simulink model "EPLL_PFC"  (R2019b)
settings: Solver=ode45  StartTime=0.0  StopTime=1  MaxStep=1e-6  AbsTol=1e-6
values from neighbouring files (symbols this model uses):
  C = 4000e-6    (= 0.004)    [EPLL_PFC_params.m]
  E = 670    [EPLL_PFC_params.m]
  f_VT = 3700    [EPLL_PFC_params.m]
  K_vco = 1    [EPLL_PFC_params.m]
  L = (400e-6)/2    (= 0.0002)    [EPLL_PFC_params.m]
  mu_1 = 200    [EPLL_PFC_params.m]
  omega_vco_free = 50 * 2 * pi    (= 314.159265359)    [EPLL_PFC_params.m]
  R = 1.22    [EPLL_PFC_params.m]
  t_step = 1/f_VT/N1    (= 1.35135135135e-06)    [EPLL_PFC_params.m]
  tau_1 = 1/mu_2    (= 5e-05)    [EPLL_PFC_params.m]
  tau_2 = mu_3/mu_2    (= 0.02)    [EPLL_PFC_params.m]
undefined symbols (not defined in the file or in its folder): sawtooth
libraries: powerlib x15
settings Model: Creator=Vogal  LastModifiedBy=mir
settings SolverCC: AutoScaleAbsTol=off  InitialStep=1e-6
settings DataIOCC: ReturnWorkspaceOutputs=off
settings OptimizationCC: LifeSpan=inf
settings DebuggingCC: AllowSymbolicDim=off  SFExecutionAtInitializationDiag=none  ArithmeticOperatorsInVariantConditions=warning
settings HardwareCC: ProdBitPerSizeT=32  ProdBitPerPtrDiffT=32  ProdWordSize=32  ProdHWDeviceType=Specified
settings SFSimCC: SimUseLocalCustomCode=off  CustomCodeUndefinedFunction=UseInterfaceOnly
settings RTWCC: RTWUseLocalCustomCode=off
settings CodeAppCC: StateflowObjectComments=on
settings SimscapeCC: SimscapeNormalizeSystem=off

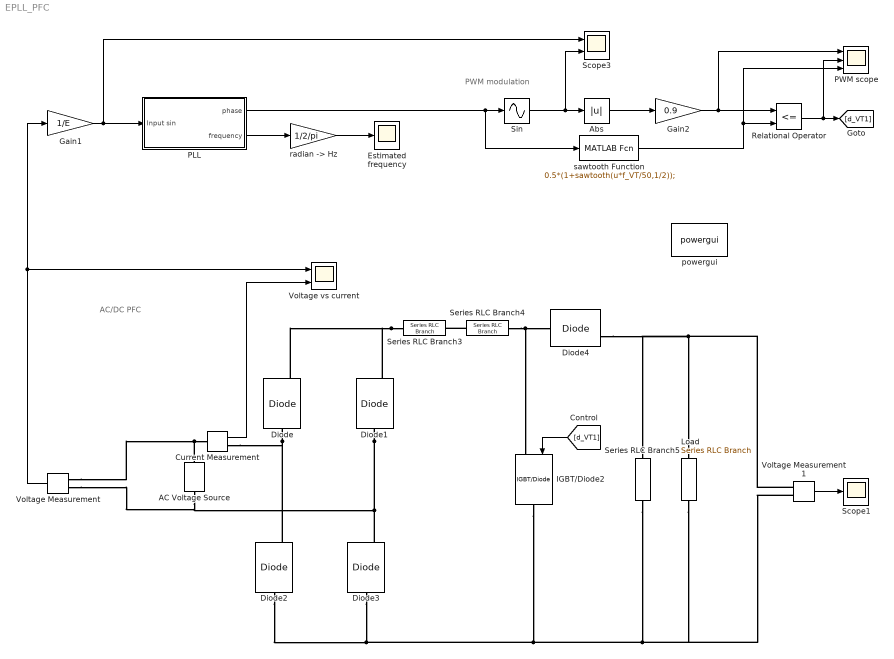
== system EPLL_PFC ==
  note: PWM modulation
  note: AC/DC PFC
  AC Voltage Source : powerlib/Electrical Sources/AC Voltage Source  Amplitude=E  Phase=0  Frequency=55  SampleTime=0  Measurements=None  BusType=swing  Pref=10e3  Qref=0  Qmin=-inf  Qmax=+inf
      settings: SourceProductName=Simscape Electrical
  Abs : Abs
  Current Measurement : powerlib/Measurements/Current Measurement  PhasorSimulation=off  OutputType=Complex  PSBequivalent=0
      settings: SourceProductName=Simscape Electrical
  Diode{,1..4} (5 alike) : powerlib/Power Electronics/Diode  Ron=0.001  Lon=0  Vf=0.8  IC=0  UseSnubber=off  Rs=500  Cs=250e-9  Measurements=on
      settings: SourceProductName=Simscape Electrical
  Estimated frequency : Scope
  Gain1 : Gain  Gain=1/E
  Gain2 : Gain  Gain=0.9
  IGBT/Diode2 : powerlib/Power Electronics/IGBT//Diode  Ron=1e-3  Rs=1e5  Cs=inf  Measurements=off
      settings: SourceProductName=Simscape Electrical
  Load : powerlib/Elements/Series RLC Branch  LConnTagsString=__new0  RConnTagsString=__new0  BranchType=R  Resistance=R  Inductance=L  SetiL0=off  InitialCurrent=0  Capacitance=C  Setx0=off  InitialVoltage=0  Measurements=None
      settings: SourceProductName=Simscape Electrical
  PLL : Subsystem
  PWM scope : Scope  NumInputPorts=3
  Relational Operator : RelationalOperator  Operator=<=  OutDataTypeStr=boolean  RndMeth=Nearest
  Scope1 : Scope
  Scope3 : Scope  NumInputPorts=2
  Series RLC Branch3 : powerlib/Elements/Series RLC Branch  LConnTagsString=__new0  RConnTagsString=__new0  BranchType=L  Resistance=R  Inductance=L  SetiL0=off  InitialCurrent=0  Capacitance=1e-6  Setx0=off  InitialVoltage=0  Measurements=None
      settings: SourceProductName=Simscape Electrical
  Series RLC Branch4 : powerlib/Elements/Series RLC Branch  LConnTagsString=__new0  RConnTagsString=__new0  BranchType=R  Resistance=1  Inductance=L  SetiL0=off  InitialCurrent=0  Capacitance=C  Setx0=off  InitialVoltage=0  Measurements=None
      settings: SourceProductName=Simscape Electrical
  Series RLC Branch5 : powerlib/Elements/Series RLC Branch  LConnTagsString=__new0  RConnTagsString=__new0  BranchType=C  Resistance=R  Inductance=L  SetiL0=off  InitialCurrent=0  Capacitance=C  Setx0=off  InitialVoltage=0  Measurements=None
      settings: SourceProductName=Simscape Electrical
  Sin : Sin  TimeSource=Use external signal  SampleTime=0
  Voltage Measurement : powerlib/Measurements/Voltage Measurement  PhasorSimulation=off  OutputType=Complex  PSBequivalent=0
      settings: SourceProductName=Simscape Electrical
  Voltage Measurement1 : powerlib/Measurements/Voltage Measurement  PhasorSimulation=off  OutputType=Complex  PSBequivalent=0
      settings: SourceProductName=Simscape Electrical
  Voltage vs current : Scope  NumInputPorts=2
  powergui : powerlib/powergui  Priority=1  SimulationMode=Discrete  SampleTime=t_step  frequency=60  Iterations=50  frequencyindice=0  Pbase=100e6  ErrMax=1e-4  UnitsV=kV  UnitsW=MW  buscounter=0  FunctionMessages=off  echomessages=off  EnableUseOfTLC=off  CurrentSourceSwitches=off  DisableSnubberDevices=off  DisableRonSwitches=off  DisableVfSwitches=off  DisplayEquations=off  AutomaticDiscreteSolvers=off  SolverType=Tustin/Backward Euler (TBE)  Interpol=off  ExternalGateDelay=off  methode=off  Ts=10  x0status=blocks  SPID=off  SwTol=0  HookPort=off  NonlinearTolerance=1e-4  nMaxIteration=100  ContinueOnMaxIteration=off  RestoreLinks=warning  ResistiveCurrentMeasurement=off  Frange=[0:2:500]  Ylog=off  Xlog=on  ShowGrid=off  save=off  variable=ZData  structure=0  ZoomFFT=off  StartTime=0.0  cycles=1  DisplayStyle=1  fundamental=60  FreqAxis=off  MaxFrequency=1000  frequencyindicesteady=1  RmsSteady=1  display=off
      settings: SourceProductName=Simscape Electrical
  "radian -> Hz" : Gain  Gain=1/2/pi
  sawtooth Function : MATLABFcn  MATLABFcn=0.5*(1+sawtooth(u*f_VT/50,1/2));
  wires:
  [d_VT1] -> IGBT/Diode2/1
  Voltage Measurement/1 -> Gain1/1, Voltage vs current/1
  Relational Operator/1 -> PWM scope/2, [d_VT1]
  Gain2/1 -> PWM scope/1, Relational Operator/1
  Current Measurement/1 -> Voltage vs current/2
  Voltage Measurement1/1 -> Scope1/1
  Abs/1 -> Gain2/1
  Gain1/1 -> Scope3/1, PLL/1("Input sin ")
  PLL/1(phase) -> sawtooth Function/1, Sin/1
  sawtooth Function/1 -> PWM scope/3, Relational Operator/2
  PLL/2(frequency) -> "radian -> Hz"/1
  "radian -> Hz"/1 -> Estimated frequency/1
  Sin/1 -> Scope3/2, Abs/1
  connections:
  Diode3/LConn1 -- Diode2/LConn1 -- Load/RConn1 -- Voltage Measurement1/LConn2 -- Series RLC Branch5/RConn1 -- IGBT/Diode2/RConn1
  Diode/LConn1 -- Diode2/RConn1 -- Current Measurement/RConn1
  Series RLC Branch5/LConn1 -- Diode4/RConn1 -- Load/LConn1 -- Voltage Measurement1/LConn1
  Series RLC Branch4/LConn1 -- IGBT/Diode2/LConn1 -- Diode4/LConn1
  Series RLC Branch3/LConn1 -- Diode/RConn1 -- Diode1/RConn1
  Diode1/LConn1 -- Voltage Measurement/LConn2 -- AC Voltage Source/LConn1 -- Diode3/RConn1
  Series RLC Branch4/RConn1 -- Series RLC Branch3/RConn1
  AC Voltage Source/RConn1 -- Voltage Measurement/LConn1 -- Current Measurement/LConn1

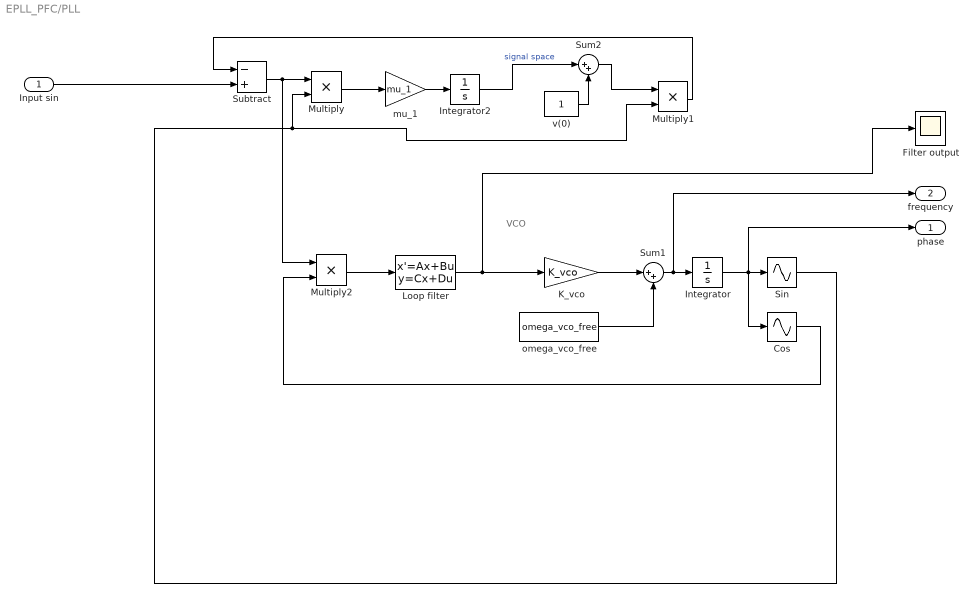
== system EPLL_PFC/PLL ==
  note: VCO
  "Input sin " : Inport
  Cos : Sin  TimeSource=Use external signal  Phase=pi/2  SampleTime=0
  Filter output : Scope
  Integrator : Integrator
  Integrator2 : Integrator
  K_vco : Gain  Gain=K_vco
  Loop filter : StateSpace  A=0  B=u/2/tau_1  D=tau_2*u/2/tau_1  InitialCondition=0
  Multiply : Product
  Multiply1 : Product
  Multiply2 : Product
  Sin : Sin  TimeSource=Use external signal  SampleTime=0
  Subtract : Sum  Inputs=-+
  Sum1 : Sum  Inputs=|++
  Sum2 : Sum  Inputs=|++
  mu_1 : Gain  Gain=mu_1
  omega_vco_free : Constant  Value=omega_vco_free
  v(0) : Constant
  phase : Outport
  frequency : Outport  Port=2
  wires:
  "Input sin "/1 -> Subtract/2
  Multiply1/1 -> Subtract/1
  K_vco/1 -> Sum1/1
  omega_vco_free/1 -> Sum1/2
  Cos/1 -> Multiply2/2
  Integrator/1 -> phase/1, Cos/1, Sin/1
  Subtract/1 -> Multiply2/1, Multiply/1
  Sum1/1 -> frequency/1, Integrator/1
  Loop filter/1 -> Filter output/1, K_vco/1
  mu_1/1 -> Integrator2/1
  Sin/1 -> Multiply1/2, Multiply/2
  Multiply/1 -> mu_1/1
  Multiply2/1 -> Loop filter/1
  Integrator2/1 -> Sum2/1  "signal space"
  Sum2/1 -> Multiply1/1
  v(0)/1 -> Sum2/2
